simulink model "hw2_p8_c"  (R2020a)
settings: Solver=VariableStepAuto  StartTime=0.0  StopTime=20  RelTol=1e-3
settings Model: Creator=Tomo  LastModifiedBy=Tomo

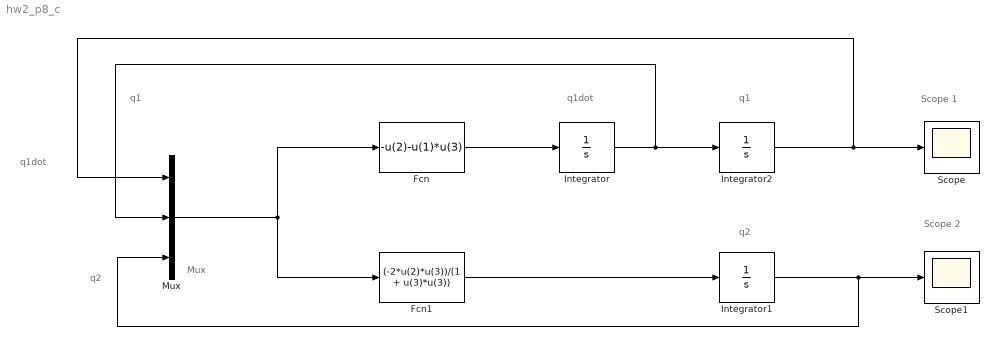
== system hw2_p8_c ==
  note: Scope 1
  note: Mux
  note: q1dot
  note: q1
  note: q2
  note: Scope 2
  note: q1
  note: q1dot
  note: q2
  Fcn : Fcn  Expr=-u(2)-u(1)*u(3)
  Fcn1 : Fcn  Expr=(-2*u(2)*u(3))/(1 + u(3)*u(3))
  Integrator : Integrator
  Integrator1 : Integrator  InitialCondition=0.5
  Integrator2 : Integrator  InitialCondition=0.2
  Mux : Mux  Inputs=3
  Scope : Scope
  Scope1 : Scope
  wires:
  Fcn1/1 -> Integrator1/1
  Integrator1/1 -> Mux/3, Scope1/1
  Fcn/1 -> Integrator/1
  Integrator/1 -> Integrator2/1, Mux/2
  Mux/1 -> Fcn1/1, Fcn/1
  Integrator2/1 -> Mux/1, Scope/1
